simulink model "BD_CONV2"  (Simulink 4.1.1)
settings: Solver=ode1  SolverMode=SingleTasking  StartTime=0.0  StopTime=max(cyc_mph(:,1))  FixedStep=1  MaxStep=1  RelTol=1e-3  AbsTol=1e-3
undefined symbols (not defined in the file): cyc_mph, ess_on, ex_calc, fc_ct_trq, fc_emis, fc_inertia, fc_map_spd, fc_max_trq, fc_spd_scale, fc_trq_scale, fd_inertia, fd_loss, fd_ratio, gb_dnshift_load, gb_dnshift_spd, gb_gears_num, gb_inertia, gb_num_init, gb_ratio, gb_shift_delay, gb_spd_scale, gb_trq_scale, gb_upshift_load, gb_upshift_spd, logFlag, tx_eff_map, tx_map_spd, tx_map_trq, vc_clutch_bool, vc_idle_bool, vc_idle_spd, vc_key_on, vc_launch_spd, veh_air_density, veh_CD, veh_FA, veh_gravity, veh_mass, wh_axle_loss_mass, wh_axle_loss_trq, wh_front_active_bool, wh_inertia, wh_max_front_brake_force, wh_max_rear_brake_force, wh_radius, wh_rear_active_bool, wh_slip, wh_slip_force_coeff
libraries: lib_wheel2 x12, lib_drive_cycle2 x2, lib_accessory2 x2, lib_etc x2, lib_interactive x1, lib_exhaust x1, lib_fuel_converter3 x1, lib_help x1
(part 11 of 11)

== system BD_CONV2/<cs> control strategy/Clutch Control/Clutch Control/clutch control/gearbox speed estimator ==
  gb_spd_in_r if no gear change : Inport  Port=1  LatchInput=off
  Block NOTES : Subsystem
      settings: RTWFcnNameOpts=Auto  RTWFileNameOpts=Auto
      mask Display: disp('Block\nNOTES')
  Constant : Constant  Orientation=left  Value=eps
  Constant1 : Constant  Orientation=left  Value=0
  Constant2 : Constant  Orientation=left  Value=1
  Constant3 : Constant  Orientation=left  Value=0.11
  Gain : Gain  Gain=0.447  Multiplication=Element-wise(K.*u)  SaturateOnIntegerOverflow=on
  IC : InitialCondition  Value=cyc_mph(1,2)*0.447/wh_radius*fd_ratio*gb_ratio(gb_num_init)
  IC1 : InitialCondition  Value=1
  Logical : Logic  Operator=AND  Inputs=2
  Product : Product  Inputs=**/  Multiplication=Element-wise(.*)  SaturateOnIntegerOverflow=on
  Relational : RelationalOperator  Operator=>
  Relational1 : RelationalOperator  Operator=<=
  Sum : Sum  Inputs=++  SaturateOnIntegerOverflow=on
  Sum1 : Sum  Inputs=-+  SaturateOnIntegerOverflow=on
  Switch : Switch  Threshold=eps
  Switch1 : Switch  Threshold=eps
  dt : Subsystem
      settings: RTWFcnNameOpts=Auto  RTWFileNameOpts=Auto
  Out1 : Outport  Port=1
  wires:
  dt/1(Out1) -> Relational1/1
  Logical/1 -> Switch1/2
  IC1/1 -> Logical/1
  Relational1/1 -> Logical/2
  Constant3/1 -> Relational1/2
  [gb_spd_in_a] -> Product/1
  gb_spd_in_r if no gear change/1 -> Switch1/3
  Switch1/1 -> Out1/1
  Switch/1 -> IC/1
  Relational/1 -> IC1/1
  Sum1/1 -> Relational/1
  Constant2/1 -> Relational/2
  [mpha] -> Sum1/1, Gain/1
  [cyc_mph_r] -> Sum1/2
  Constant/1 -> Sum/2
  IC/1 -> Switch1/1
  Constant1/1 -> Switch/3
  [veh_spd_a_rec] -> Switch/2, Sum/1
  Gain/1 -> Product/2
  Sum/1 -> Product/3
  Product/1 -> Switch/1

== system BD_CONV2/<cs> control strategy/Fuel Converter Control conventional ic engine/conventional IC engine/Fuel Converter Control/key_on ==
  Clock : Clock
      settings: DisplayTime=off  Decimation=10
  Fcn1 : Fcn  Expr=rem(u[1],period)
  Look-Up Table : Lookup  InputValues=t  OutputValues=y
  out_1 : Outport  Port=1  InitialOutput=0
  wires:
  Fcn1/1 -> Look-Up Table/1
  Clock/1 -> Fcn1/1
  Look-Up Table/1 -> out_1/1

== system BD_CONV2/<cs> control strategy/Gearbox Control manual shift logic/manual shift logic/gearbox  control/Block NOTES ==
  note: This gearbox control block computes the current gear number given the gearbox's
      | req'd output torque and speed and an estimate its efficiency.  Upshifts occur, given a
      | certain engine speed,  when the estimated engine load falls below the upshift curve
      | in engine speed/load space, and downshifts likewise occur when estimated engine
      | load rises above the downshift curve.  Separate upshift and downshift curves are
      | defined for each gear.  An upshift may not be immediately followed by a downshift.
      | If the tires are about to slip, don't upshift unless the engine would be at max. speed.
      | Enforce this rule by setting the load to 1 when the tires are about to slip.

== system BD_CONV2/<cs> control strategy/Gearbox Control manual shift logic/manual shift logic/gearbox  control/allow downshift? ==
  prev gearnum : Inport  Port=1  LatchInput=off
  Logical Operator : Logic  Operator=NOR  Inputs=2
  Memory : Memory  X0=1  InheritSampleTime=off
      settings: RTWStateStorageClass=Auto
  Memory1 : Memory  X0=1  InheritSampleTime=off
      settings: RTWStateStorageClass=Auto
  Relational Operator1 : RelationalOperator  Operator=>
  Relational Operator2 : RelationalOperator  Operator=>
  allow shift : Outport  Port=1  InitialOutput=0
  wires:
  Logical Operator/1 -> allow shift/1
  prev gearnum/1 -> Relational Operator1/1, Memory/1, Relational Operator2/1
  Relational Operator1/1 -> Logical Operator/1
  Memory/1 -> Relational Operator1/2, Memory1/1
  Memory1/1 -> Relational Operator2/2
  Relational Operator2/1 -> Logical Operator/2

== system BD_CONV2/<cs> control strategy/Gearbox Control manual shift logic/manual shift logic/gearbox  control/downshift  command ==
  prev gear number : Inport  Port=1  LatchInput=off
  engine load : Inport  Port=2  LatchInput=off
  engine speed : Inport  Port=3  LatchInput=off
  Mux : Mux  Inputs=2
      settings: DisplayOption=none
  Relational Operator : RelationalOperator  Operator=>
  load fraction : Subsystem  mask(Gear Selector){spd=gb_dnshift_spd, load=gb_dnshift_load}
      mask prompts: spd "Speeds:"; load "Load Fractions:"
      mask help:
      | This block will perform a linear interplation (extrapolation outside of bounds) to determine the shift point load fraction associated with the current gear number and speed.
      |
      | The Speeds parameter should be defined as an array of vectors containing speeds for each gear number.  The Load Fractions parameter should be defined as a array of vectors containing load fractions indexed by the speeds in the Speeds parameter for each gear number.
      settings: RTWFcnNameOpts=Auto  RTWFileNameOpts=Auto
      mask Help:
      | Reference the base workspace variables - gb_**shift_spd and gb_**shift_load  where ** is either up for upshift conditions or dn for downshift conditions.
      | 
      | Or define the arrays as follows:
      | 
      | {[spd1 spd2 spd3 spd4]; [spd1 spd2 spd3 spd4]; ...}
      | 
      | {[load1 load2 load3 load4]; [load1 load2 load3 load4]; ...}
      | 
      | where each array contains one row for each gear in the gearbox.  Speeds should be defined in rad/s and loads as a decimal fraction.
  command : Outport  Port=1  InitialOutput=0
  wires:
  load fraction/1(Out1) -> Relational Operator/2
  Mux/1 -> load fraction/1(In1)
  engine load/1 -> Relational Operator/1
  prev gear number/1 -> Mux/1
  engine speed/1 -> Mux/2
  Relational Operator/1 -> command/1

== system BD_CONV2/<cs> control strategy/Gearbox Control manual shift logic/manual shift logic/gearbox  control/gearbox speed estimator ==
  gb_spd_in_r if no gear change : Inport  Port=1  LatchInput=off
  Block NOTES : Subsystem
      settings: RTWFcnNameOpts=Auto  RTWFileNameOpts=Auto
      mask Display: disp('Block\nNOTES')
  Constant : Constant  Orientation=left  Value=eps
  Constant1 : Constant  Orientation=left  Value=0
  Constant2 : Constant  Orientation=left  Value=1
  Constant3 : Constant  Orientation=left  Value=0.11
  Gain : Gain  Gain=0.447  Multiplication=Element-wise(K.*u)  SaturateOnIntegerOverflow=on
  IC : InitialCondition  Value=cyc_mph(1,2)*0.447/wh_radius*fd_ratio*gb_ratio(gb_num_init)
  IC1 : InitialCondition  Value=1
  Logical : Logic  Operator=AND  Inputs=2
  Product : Product  Inputs=**/  Multiplication=Element-wise(.*)  SaturateOnIntegerOverflow=on
  Relational : RelationalOperator  Operator=>
  Relational1 : RelationalOperator  Operator=<=
  Sum : Sum  Inputs=++  SaturateOnIntegerOverflow=on
  Sum1 : Sum  Inputs=-+  SaturateOnIntegerOverflow=on
  Switch : Switch  Threshold=eps
  Switch1 : Switch  Threshold=eps
  dt : Subsystem
      settings: RTWFcnNameOpts=Auto  RTWFileNameOpts=Auto
  Out1 : Outport  Port=1
  wires:
  Product/1 -> Switch/1
  Sum/1 -> Product/3
  Gain/1 -> Product/2
  [veh_spd_a_rec] -> Sum/1, Switch/2
  Constant1/1 -> Switch/3
  IC/1 -> Switch1/1
  Constant/1 -> Sum/2
  [cyc_mph_r] -> Sum1/2
  [mpha] -> Gain/1, Sum1/1
  Constant2/1 -> Relational/2
  Sum1/1 -> Relational/1
  Relational/1 -> IC1/1
  Switch/1 -> IC/1
  Switch1/1 -> Out1/1
  gb_spd_in_r if no gear change/1 -> Switch1/3
  [gb_spd_in_a] -> Product/1
  Constant3/1 -> Relational1/2
  Relational1/1 -> Logical/2
  IC1/1 -> Logical/1
  Logical/1 -> Switch1/2
  dt/1(Out1) -> Relational1/1

== system BD_CONV2/<cs> control strategy/Gearbox Control manual shift logic/manual shift logic/gearbox  control/shifting1 ==
  gear number : Inport  Port=1  LatchInput=off
  Constant : Constant  Value=gb_shift_delay-1e-6
  Relational Operator : RelationalOperator  Operator=<
  time since last shift : Subsystem
      settings: RTWFcnNameOpts=Auto  RTWFileNameOpts=Auto
      mask Display: disp('time since\nlast shift')
  out_1 : Outport  Port=1  InitialOutput=0
  wires:
  Relational Operator/1 -> out_1/1
  gear number/1 -> time since last shift/1(in_1)
  Constant/1 -> Relational Operator/2
  time since last shift/1(out_1) -> Relational Operator/1

== system BD_CONV2/<cs> control strategy/Gearbox Control manual shift logic/manual shift logic/gearbox  control/upshift  command ==
  prev gear number : Inport  Port=1  LatchInput=off
  engine load : Inport  Port=2  LatchInput=off
  engine speed : Inport  Port=3  LatchInput=off
  Mux : Mux  Inputs=2
      settings: DisplayOption=none
  Relational Operator : RelationalOperator  Operator=<
  load fraction : Subsystem  mask(Gear Selector){spd=gb_upshift_spd, load=gb_upshift_load}
      mask prompts: spd "Speeds:"; load "Load Fractions:"
      mask help:
      | This block will perform a linear interplation (extrapolation outside of bounds) to determine the shift point load fraction associated with the current gear number and speed.
      |
      | The Speeds parameter should be defined as an array of vectors containing speeds for each gear number.  The Load Fractions parameter should be defined as a array of vectors containing load fractions indexed by the speeds in the Speeds parameter for each gear number.
      settings: RTWFcnNameOpts=Auto  RTWFileNameOpts=Auto
      mask Help:
      | Reference the base workspace variables - gb_**shift_spd and gb_**shift_load  where ** is either up for upshift conditions or dn for downshift conditions.
      | 
      | Or define the arrays as follows:
      | 
      | {[spd1 spd2 spd3 spd4]; [spd1 spd2 spd3 spd4]; ...}
      | 
      | {[load1 load2 load3 load4]; [load1 load2 load3 load4]; ...}
      | 
      | where each array contains one row for each gear in the gearbox.  Speeds should be defined in rad/s and loads as a decimal fraction.
  command : Outport  Port=1  InitialOutput=0
  wires:
  load fraction/1(Out1) -> Relational Operator/2
  engine load/1 -> Relational Operator/1
  prev gear number/1 -> Mux/1
  Mux/1 -> load fraction/1(In1)
  engine speed/1 -> Mux/2
  Relational Operator/1 -> command/1

== system BD_CONV2/ACC MECH <accm>/mechanical accessory model and interface/Mechanical Accessory model/backward model/enhancedToWorkspace ==
  In1 : Inport  Port=1  LatchInput=off
  To Workspace : ToWorkspace  VariableName=acc_mech_pwr_r  SampleTime=-1  SaveFormat=Array
  wires:
  In1/1 -> To Workspace/1

== system BD_CONV2/ACC MECH <accm>/mechanical accessory model and interface/Mechanical Accessory model/backward model/enhancedToWorkspace1 ==
  In1 : Inport  Port=1  LatchInput=off
  To Workspace : ToWorkspace  VariableName=acc_mech_trq_r  SampleTime=-1  SaveFormat=Array
  wires:
  In1/1 -> To Workspace/1

== system BD_CONV2/ACC MECH <accm>/mechanical accessory model and interface/Mechanical Accessory model/backward model/mechanical accessories (Nm) ==
  w_APU : Inport  Port=1  LatchInput=off
  Mechanical Accessories: Const Mech Var Elect : lib_accessory2/ACC MECH models/Mechanical Accessories: Const Mech Var Elect
  T_acc : Outport  Port=1
  P_mech_acc : Outport  Port=2
  wires:
  w_APU/1 -> Mechanical Accessories: Const Mech Var Elect/1
  Mechanical Accessories: Const Mech Var Elect/1 -> T_acc/1
  Mechanical Accessories: Const Mech Var Elect/2 -> P_mech_acc/1

== system BD_CONV2/fuel converter <fc>/IC Engine Model  &  Interface/ic engine model/engine speed estimator/Block NOTES ==
  note: If the clutch is engaged and the trace was missed in the previous time step:
      | The estimated engine speed for the current time step is the actual engine
      | speed from the previous time step.
      |
      | If the clutch is disengaged and the speed is commanded to increase (spin up):
      | The engine speed is the lesser of the commanded speed and the maximum
      | speed attainable given the engine capability.
      |
      | If the clutch is disengaged at the speed is commanded to decrease (spin down):
      | The engine speed is computed by integrating with respect to time the ratio of
      |  closed-throttle torque to engine inertia.
      |
      | Otherwise:
      | The engine speed is equal to the speed command, but no greater than the
      | engine's maximum speed nor less than the engine's idle speed (if the engine is on.)

== system BD_CONV2/fuel converter <fc>/IC Engine Model  &  Interface/ic engine model/engine speed estimator/dt ==
  Clock : Clock
      settings: DisplayTime=off  Decimation=10
  Memory1 : Memory  X0=-0.1  InheritSampleTime=off
      settings: RTWStateStorageClass=Auto
  Sum1 : Sum  Inputs=+-  SaturateOnIntegerOverflow=on
  out_1 : Outport  Port=1  InitialOutput=0
  wires:
  Clock/1 -> Sum1/1, Memory1/1
  Memory1/1 -> Sum1/2
  Sum1/1 -> out_1/1

== system BD_CONV2/fuel converter <fc>/IC Engine Model  &  Interface/ic engine model/engine speed estimator/effect of inertia (Nm) ==
  req'd spd (rad/s) : Inport  Port=1  LatchInput=off
  prev spd : Inport  Port=2  LatchInput=off
  Clock : Clock
      settings: DisplayTime=off  Decimation=10
  Constant : Constant  Value=fc_inertia
  Memory : Memory  X0=-0.1  InheritSampleTime=off
      settings: RTWStateStorageClass=Auto
  Product1 : Product  Inputs=**/  Multiplication=Element-wise(.*)  SaturateOnIntegerOverflow=on
  Sum : Sum  Inputs=+-  SaturateOnIntegerOverflow=on
  Sum1 : Sum  Inputs=+-  SaturateOnIntegerOverflow=on
  (Nm) : Outport  Port=1  InitialOutput=0
  wires:
  Constant/1 -> Product1/1
  Clock/1 -> Sum1/1, Memory/1
  Memory/1 -> Sum1/2
  Product1/1 -> (Nm)/1
  prev spd/1 -> Sum/2
  req'd spd (rad/s)/1 -> Sum/1
  Sum1/1 -> Product1/3
  Sum/1 -> Product1/2

== system BD_CONV2/fuel converter <fc>/IC Engine Model  &  Interface/ic engine model/engine speed estimator/just started spin-down/spin-up ==
  state : Inport  Port=1  LatchInput=off
  Logical Operator : Logic  Operator=AND  Inputs=2
  Logical Operator1 : Logic  Operator=NOT  Inputs=1
  Memory1 : Memory  X0=1  InheritSampleTime=off
      settings: RTWStateStorageClass=Auto
  trigger : Outport  Port=1  InitialOutput=0
  wires:
  state/1 -> Memory1/1, Logical Operator/1
  Logical Operator/1 -> trigger/1
  Logical Operator1/1 -> Logical Operator/2
  Memory1/1 -> Logical Operator1/1

== system BD_CONV2/fuel converter <fc>/IC Engine Model  &  Interface/ic engine model/engine speed estimator/no-lag Reset Integrator ==
  in_1 : Inport  Port=1  LatchInput=off
  in_2 : Inport  Port=2  LatchInput=off
  in_3 : Inport  Port=3  LatchInput=off
  Constant : Constant  Value=0
  Memory : Memory  Orientation=left  X0=initval  InheritSampleTime=off
      settings: RTWStateStorageClass=Auto
  Product : Product  Inputs=2  Multiplication=Element-wise(.*)  SaturateOnIntegerOverflow=on
  Sum : Sum  Inputs=++  SaturateOnIntegerOverflow=on
  Switch : Switch  Threshold=eps
  dt : Subsystem  Orientation=down
      settings: RTWFcnNameOpts=Auto  RTWFileNameOpts=Auto
  in_2==0 : RelationalOperator  Operator===
  out_1 : Outport  Port=1  InitialOutput=0
  wires:
  Constant/1 -> in_2==0/2
  in_2==0/1 -> Switch/2
  Switch/1 -> Memory/1, out_1/1
  Sum/1 -> Switch/1
  Memory/1 -> Sum/1
  Product/1 -> Sum/2
  dt/1(out_1) -> Product/1
  in_1/1 -> Product/2
  in_2/1 -> in_2==0/1
  in_3/1 -> Switch/3

== system BD_CONV2/fuel converter <fc>/IC Engine Model  &  Interface/ic engine model/engine torque/Block NOTES ==
  note: If the engine is not spinning down with the clutch disengaged:
      | 1.  Engine brake (aka map) torque is given by the required shaft
      | torque plus enough torque to accelerate the engine's rotating
      | parts as commanded and torque to power the accessories,
      | subject to the engine's torque limits at the current speed.
      | 2.  Shaft torque is engine brake torque less the effects of inertia
      | and accessories.
      |
      | If the engine is spinning down:
      | 1.  Engine brake/map torque is the closed-throttle torque.
      | 2.  Shaft torque is zero.

== system BD_CONV2/fuel converter <fc>/IC Engine Model  &  Interface/ic engine model/engine torque/T_closed throttle ==
  w_APU : Inport  Port=1  LatchInput=off
  Saturation : Saturate  UpperLimit=max(fc_map_spd)*fc_spd_scale  LowerLimit=min(fc_map_spd)*fc_spd_scale  LinearizeAsGain=on
  ctt lookup : Lookup  InputValues=fc_map_spd*fc_spd_scale  OutputValues=fc_ct_trq*fc_trq_scale
  T_closed throttle : Outport  Port=1  InitialOutput=0
  wires:
  ctt lookup/1 -> T_closed throttle/1
  Saturation/1 -> ctt lookup/1
  w_APU/1 -> Saturation/1

== system BD_CONV2/fuel converter <fc>/IC Engine Model  &  Interface/ic engine model/engine torque/T_max ==
  w_APU : Inport  Port=1  LatchInput=off
  Saturation1 : Saturate  UpperLimit=max(fc_map_spd)*fc_spd_scale  LowerLimit=min(fc_map_spd)*fc_spd_scale  LinearizeAsGain=on
  max_torque lookup : Lookup  InputValues=fc_map_spd*fc_spd_scale  OutputValues=fc_max_trq*fc_trq_scale
  T_max : Outport  Port=1  InitialOutput=0
  tag scope: engine_speed=scoped
  wires:
  w_APU/1 -> Saturation1/1
  max_torque lookup/1 -> T_max/1
  Saturation1/1 -> max_torque lookup/1, [engine_speed]

== system BD_CONV2/fuel converter <fc>/IC Engine Model  &  Interface/ic engine model/engine torque/effect of inertia (Nm) ==
  engine spd (rad/s) : Inport  Port=1  LatchInput=off
  >=0 : Saturate  UpperLimit=inf  LowerLimit=0  LinearizeAsGain=on
  Block NOTES : Subsystem
      settings: RTWFcnNameOpts=Auto  RTWFileNameOpts=Auto
      mask Display: disp('Block\nNOTES')
  Clock : Clock
      settings: DisplayTime=off  Decimation=10
  Constant : Constant  Orientation=left  Value=fc_inertia
  Constant1 : Constant  Value=max(fc_max_trq)*fc_trq_scale
  Constant2 : Constant  Orientation=left  Value=0.01
  Memory : Memory  X0=-0.1  InheritSampleTime=off
      settings: RTWStateStorageClass=Auto
  Memory1 : Memory  X0=vc_idle_spd*vc_key_on(1,2)  InheritSampleTime=off
      settings: RTWStateStorageClass=Auto
  MinMax : MinMax  Function=min  Inputs=2
  Product : Product  Inputs=2  Multiplication=Element-wise(.*)  SaturateOnIntegerOverflow=on
  Product1 : Product  Inputs=*/*  Multiplication=Element-wise(.*)  SaturateOnIntegerOverflow=on
  Relational : RelationalOperator  Operator=>
  Sum : Sum  Inputs=+-  SaturateOnIntegerOverflow=on
  Sum1 : Sum  Inputs=+-  SaturateOnIntegerOverflow=on
  Sum2 : Sum  Inputs=-+  SaturateOnIntegerOverflow=on
  Switch : Switch  Threshold=eps
  engine inertia as a function of total vehicle inertia (generous approximation) : Subsystem  Orientation=down
      settings: RTWFcnNameOpts=Auto  RTWFileNameOpts=Auto
  (Nm) : Outport  Port=1  InitialOutput=0
  wires:
  Sum/1 -> >=0/1, Switch/3
  Memory1/1 -> Sum/2
  Product/1 -> MinMax/1
  Constant1/1 -> Product/2
  engine inertia as a function of total vehicle inertia (generous approximation)/1(Out1) -> Product/1
  Product1/1 -> MinMax/2
  MinMax/1 -> (Nm)/1
  [cyc_mph_r_prev] -> Sum2/2
  [mpha_prev] -> Sum2/1
  Switch/1 -> Product1/1
  Sum1/1 -> Product1/2
  Constant/1 -> Product1/3
  Memory/1 -> Sum1/2
  Clock/1 -> Memory/1, Sum1/1
  Relational/1 -> Switch/2
  >=0/1 -> Switch/1
  Sum2/1 -> Relational/1
  Constant2/1 -> Relational/2
  engine spd (rad/s)/1 -> Memory1/1, Sum/1

== system BD_CONV2/gearbox <gb> old/gearbox model & interface/gearbox model/Pout/Pin neglecting inertia/Pout/Pin (neglecting inertia) ==
  in_1 : Inport  Port=1  LatchInput=off
  in_2 : Inport  Port=2  LatchInput=off
  Fcn : Fcn  Expr=1/u
  Product : Product  Inputs=2  Multiplication=Element-wise(.*)  SaturateOnIntegerOverflow=on
  out_1 : Outport  Port=1  InitialOutput=0
  wires:
  in_1/1 -> Product/1
  Fcn/1 -> Product/2
  Product/1 -> out_1/1
  in_2/1 -> Fcn/1

== system BD_CONV2/gearbox <gb> old/gearbox model & interface/gearbox model/Pout/Pin neglecting inertia/make division bombproof ==
  note: only add eps if Tin-Tinertia is == 0 (this avoids problems when Tin-Tineratia == -eps
      | which happens from time to time
  Tin-Tinertia : Inport  Port=1  LatchInput=off
  Block NOTES : Subsystem
      settings: RTWFcnNameOpts=Auto  RTWFileNameOpts=Auto
      mask Display: disp('Block\nNOTES')
  Constant : Constant  Orientation=up  Value=eps
  Constant1 : Constant  Orientation=up  Value=0
  Product : Product  Inputs=2  Multiplication=Element-wise(.*)  SaturateOnIntegerOverflow=on
  Relational Operator1 : RelationalOperator  Operator===
  make division bombproof : Sum  Inputs=++  SaturateOnIntegerOverflow=on
  Out1 : Outport  Port=1
  wires:
  Tin-Tinertia/1 -> make division bombproof/1, Relational Operator1/1
  Constant1/1 -> Relational Operator1/2
  Product/1 -> make division bombproof/2
  Relational Operator1/1 -> Product/1
  Constant/1 -> Product/2
  make division bombproof/1 -> Out1/1

== system BD_CONV2/gearbox <gb> old/gearbox model & interface/gearbox model/gearbox controller interface/enhancedToWorkspace1 ==
  In1 : Inport  Port=1  LatchInput=off
  To Workspace : ToWorkspace  VariableName=gb_gear_ratio  SampleTime=-1  SaveFormat=Array
  wires:
  In1/1 -> To Workspace/1

== system BD_CONV2/gearbox <gb> old/gearbox model & interface/gearbox model/gearbox controller interface/enhancedToWorkspace8 ==
  In1 : Inport  Port=1  LatchInput=off
  To Workspace : ToWorkspace  VariableName=gb_shifting  SampleTime=-1  SaveFormat=Array
  wires:
  In1/1 -> To Workspace/1

== system BD_CONV2/gearbox <gb> old/gearbox model & interface/gearbox model/loss (Nm)/3D discrete lookup table (sfun) ==
  lookup speed (rad/s) : Inport  Port=1  LatchInput=off
  lookup trq (Nm) : Inport  Port=2  LatchInput=off
  "gear_number  (e.g., 1, 2, 3)" : Inport  Port=3  LatchInput=off
  Mux : Mux  Inputs=3
  Saturation : Saturate  UpperLimit=max(tx_map_spd)  LowerLimit=min(tx_map_spd)  LinearizeAsGain=on
  Saturation1 : Saturate  UpperLimit=max(tx_map_trq)  LowerLimit=min(tx_map_trq)  LinearizeAsGain=on
  Saturation2 : Saturate  UpperLimit=size(tx_eff_map,3)  LowerLimit=1  LinearizeAsGain=on
  discrete interp2d : S-Function  FunctionName=sfun_discreteLookup3d  Parameters=tx_map_trq, tx_map_spd, tx_eff_map  PortCounts=[]  SFunctionModules=''
  tx_eff : Outport  Port=1
  wires:
  Saturation2/1 -> Mux/3
  "gear_number  (e.g., 1, 2, 3)"/1 -> Saturation2/1
  Saturation1/1 -> Mux/2
  lookup trq (Nm)/1 -> Saturation1/1
  Saturation/1 -> Mux/1
  lookup speed (rad/s)/1 -> Saturation/1
  Mux/1 -> discrete interp2d/1
  discrete interp2d/1 -> tx_eff/1

== system BD_CONV2/gearbox <gb> old/gearbox model & interface/gearbox model/loss (Nm)/Block NOTES ==
  note: Revision Notes:
  note: 09/20/02:tm modifed lower input to switch after T_loss_at_input to pass the
      | total torque input as the loss when tx_eff=0
      | 5 July 2001:mpo changing loss block to a lookup table methodology
      | 12/20/00:tm revised loss saturation block. lower limit changed
      | from 1 to 0 and upper limit changed from 100 to inf to prevent over or under penalties

== system BD_CONV2/gearbox <gb> old/gearbox model & interface/gearbox model/loss (Nm)/enhancedToWorkspace ==
  In1 : Inport  Port=1  LatchInput=off
  To Workspace : ToWorkspace  VariableName=gb_current_gear_ratio  SampleTime=-1  SaveFormat=Array
  wires:
  In1/1 -> To Workspace/1

== system BD_CONV2/vehicle, wheel, & axle front/rear <wh> 2 axle --> 1 driveline/models and interface/vehicle <veh>/power logging--achieved/Joules ==
  In1 : Inport  Port=1  LatchInput=off
  To Workspace : ToWorkspace  VariableName=veh_energy_a  SampleTime=-1  SaveFormat=Array
  wires:
  In1/1 -> To Workspace/1

== system BD_CONV2/vehicle, wheel, & axle front/rear <wh> 2 axle --> 1 driveline/models and interface/vehicle <veh>/power logging--achieved/horse power ==
  In1 : Inport  Port=1  LatchInput=off
  To Workspace : ToWorkspace  VariableName=veh_pwr_a_hp  SampleTime=-1  SaveFormat=Array
  wires:
  In1/1 -> To Workspace/1

== system BD_CONV2/vehicle, wheel, & axle front/rear <wh> 2 axle --> 1 driveline/models and interface/vehicle <veh>/power logging--achieved/watts ==
  In1 : Inport  Port=1  LatchInput=off
  To Workspace : ToWorkspace  VariableName=veh_pwr_a  SampleTime=-1  SaveFormat=Array
  wires:
  In1/1 -> To Workspace/1

== system BD_CONV2/vehicle, wheel, & axle front/rear <wh> 2 axle --> 1 driveline/models and interface/vehicle <veh>/power logging--request/Joules ==
  In1 : Inport  Port=1  LatchInput=off
  To Workspace : ToWorkspace  VariableName=veh_energy_r  SampleTime=-1  SaveFormat=Array
  wires:
  In1/1 -> To Workspace/1

== system BD_CONV2/vehicle, wheel, & axle front/rear <wh> 2 axle --> 1 driveline/models and interface/vehicle <veh>/power logging--request/horse power ==
  In1 : Inport  Port=1  LatchInput=off
  To Workspace : ToWorkspace  VariableName=veh_pwr_r_hp  SampleTime=-1  SaveFormat=Array
  wires:
  In1/1 -> To Workspace/1

== system BD_CONV2/vehicle, wheel, & axle front/rear <wh> 2 axle --> 1 driveline/models and interface/vehicle <veh>/power logging--request/watts ==
  In1 : Inport  Port=1  LatchInput=off
  To Workspace : ToWorkspace  VariableName=veh_pwr_r  SampleTime=-1  SaveFormat=Array
  wires:
  In1/1 -> To Workspace/1

== system BD_CONV2/vehicle, wheel, & axle front/rear <wh> 2 axle --> 1 driveline/models and interface/vehicle <veh>/record achieved force outputs/enhancedToWorkspace ==
  In1 : Inport  Port=1  LatchInput=off
  To Workspace : ToWorkspace  VariableName=veh_pwr_accel_a  SampleTime=-1  SaveFormat=Array
  wires:
  In1/1 -> To Workspace/1

== system BD_CONV2/vehicle, wheel, & axle front/rear <wh> 2 axle --> 1 driveline/models and interface/vehicle <veh>/record achieved force outputs/enhancedToWorkspace1 ==
  In1 : Inport  Port=1  LatchInput=off
  To Workspace : ToWorkspace  VariableName=veh_pwr_drag_a  SampleTime=-1  SaveFormat=Array
  wires:
  In1/1 -> To Workspace/1

== system BD_CONV2/vehicle, wheel, & axle front/rear <wh> 2 axle --> 1 driveline/models and interface/vehicle <veh>/record achieved force outputs/enhancedToWorkspace2 ==
  In1 : Inport  Port=1  LatchInput=off
  To Workspace : ToWorkspace  VariableName=veh_pwr_ascent_a  SampleTime=-1  SaveFormat=Array
  wires:
  In1/1 -> To Workspace/1

== system BD_CONV2/vehicle, wheel, & axle front/rear <wh> 2 axle --> 1 driveline/models and interface/vehicle <veh>/record achieved force outputs/enhancedToWorkspace3 ==
  In1 : Inport  Port=1  LatchInput=off
  To Workspace : ToWorkspace  VariableName=veh_pwr_rr_a  SampleTime=-1  SaveFormat=Array
  wires:
  In1/1 -> To Workspace/1

== system BD_CONV2/vehicle, wheel, & axle front/rear <wh> 2 axle --> 1 driveline/models and interface/vehicle <veh>/record achieved force outputs/rolling resistance force ==
  average vehicle speed over time step (m/s) : Inport  Port=1  LatchInput=off
  force req'd to overcome rolling resistance (N) : lib_wheel2/Submodels/force req'd to overcome rolling resistance (N)
      settings: RTWFcnNameOpts=Auto  RTWFileNameOpts=Auto
  Fr (N) : Outport  Port=1
  wires:
  average vehicle speed over time step (m/s)/1 -> force req'd to overcome rolling resistance (N)/1
  force req'd to overcome rolling resistance (N)/1 -> Fr (N)/1

== system BD_CONV2/vehicle, wheel, & axle front/rear <wh> 2 axle --> 1 driveline/models and interface/wheel and axle  front/rear <wh>/front force/brake request  controller interface ==
  F_front_brake_req : Outport  Port=1  InitialOutput=0
  wires:
  [F_front_brake_req] -> F_front_brake_req/1

== system BD_CONV2/vehicle, wheel, & axle front/rear <wh> 2 axle --> 1 driveline/models and interface/wheel and axle  front/rear <wh>/front force/enhancedToWorkspace11 ==
  In1 : Inport  Port=1  LatchInput=off
  To Workspace : ToWorkspace  VariableName=wh_front_brake_r  SampleTime=-1  SaveFormat=Array
  wires:
  In1/1 -> To Workspace/1

== system BD_CONV2/vehicle, wheel, & axle front/rear <wh> 2 axle --> 1 driveline/models and interface/wheel and axle  front/rear <wh>/limits and losses diagnostics/enhancedToWorkspace ==
  In1 : Inport  Port=1  LatchInput=off
  To Workspace : ToWorkspace  VariableName=wh_brake_loss_pwr  SampleTime=-1  SaveFormat=Array
  wires:
  In1/1 -> To Workspace/1

== system BD_CONV2/vehicle, wheel, & axle front/rear <wh> 2 axle --> 1 driveline/models and interface/wheel and axle  front/rear <wh>/rear force/brake request controller interface1 ==
  F_rear_brake_req : Outport  Port=1  InitialOutput=0
  wires:
  [F_rear_brake_req] -> F_rear_brake_req/1

== system BD_CONV2/vehicle, wheel, & axle front/rear <wh> 2 axle --> 1 driveline/models and interface/wheel and axle  front/rear <wh>/rear force/enhancedToWorkspace ==
  In1 : Inport  Port=1  LatchInput=off
  To Workspace : ToWorkspace  VariableName=wh_rear_brake_r  SampleTime=-1  SaveFormat=Array
  wires:
  In1/1 -> To Workspace/1

== system BD_CONV2/vehicle, wheel, & axle front/rear <wh> 2 axle --> 1 driveline/models and interface/wheel and axle  front/rear <wh>/tire slip model (m/s)/Block NOTES ==
  note: This block implements the effects of finite tire slip (with respect to the road) on the
      | vehicle speed/wheel speed relationship.  Slip is defined as s=(omega*r - v) / v.  The
      | one-to-one mapping of slip to normalized tractive force, F_tract/W_front_axle, up to
      | the maximum, is stored in the variables "wh_slip" and "wh_slip_force_coeff."  The
      | slip calculation here is overridden if the actual axle speed and the requested axle
      | speed are the same, indicating that no drivetrain speed limits were encountered.

== system BD_CONV2/vehicle, wheel, & axle front/rear <wh> 2 axle --> 1 driveline/models and interface/wheel and axle  front/rear <wh>/tire slip model (m/s)/front axle ==
  In1 : Inport  Port=1  LatchInput=off
  In2 : Inport  Port=2  LatchInput=off
  Abs : Abs  SaturateOnIntegerOverflow=on
  Constant3 : Constant  Orientation=up  Value=0
  F/W : Product  Inputs=*/  Multiplication=Element-wise(.*)  SaturateOnIntegerOverflow=on
  Product : Product  Inputs=2  Multiplication=Element-wise(.*)  SaturateOnIntegerOverflow=on
  Relational Operator : RelationalOperator  Orientation=up  Operator=~=
  Saturation : Saturate  UpperLimit=max(wh_slip_force_coeff)  LowerLimit=min(wh_slip_force_coeff)  LinearizeAsGain=on
  Sign : Signum
  Switch : Switch  Threshold=0
  s=s(F/W) : Lookup  InputValues=wh_slip_force_coeff  OutputValues=wh_slip
  Out1 : Outport  Port=1
  wires:
  Product/1 -> Out1/1
  In1/1 -> F/W/2
  In2/1 -> Sign/1, Abs/1
  s=s(F/W)/1 -> Product/1
  Sign/1 -> Product/2
  F/W/1 -> Switch/1
  Switch/1 -> Saturation/1
  Saturation/1 -> s=s(F/W)/1
  Abs/1 -> Relational Operator/1, F/W/1
  Relational Operator/1 -> Switch/2
  Constant3/1 -> Relational Operator/2, Switch/3

== system BD_CONV2/vehicle, wheel, & axle front/rear <wh> 2 axle --> 1 driveline/models and interface/wheel and axle  front/rear <wh>/tire slip model (m/s)/rear axle ==
  In1 : Inport  Port=1  LatchInput=off
  In2 : Inport  Port=2  LatchInput=off
  Abs : Abs  SaturateOnIntegerOverflow=on
  Constant3 : Constant  Orientation=up  Value=0
  F/W : Product  Inputs=*/  Multiplication=Element-wise(.*)  SaturateOnIntegerOverflow=on
  Product : Product  Inputs=2  Multiplication=Element-wise(.*)  SaturateOnIntegerOverflow=on
  Relational Operator : RelationalOperator  Orientation=up  Operator=~=
  Saturation : Saturate  UpperLimit=max(wh_slip_force_coeff)  LowerLimit=min(wh_slip_force_coeff)  LinearizeAsGain=on
  Sign : Signum
  Switch : Switch  Threshold=0
  s=s(F/W) : Lookup  InputValues=wh_slip_force_coeff  OutputValues=wh_slip
  Out1 : Outport  Port=1
  wires:
  Product/1 -> Out1/1
  In1/1 -> F/W/2
  In2/1 -> Sign/1, Abs/1
  s=s(F/W)/1 -> Product/1
  Sign/1 -> Product/2
  F/W/1 -> Switch/1
  Switch/1 -> Saturation/1
  Saturation/1 -> s=s(F/W)/1
  Abs/1 -> Relational Operator/1, F/W/1
  Relational Operator/1 -> Switch/2
  Constant3/1 -> Relational Operator/2, Switch/3

== system BD_CONV2/vehicle, wheel, & axle front/rear <wh> 2 axle --> 1 driveline/models and interface/wheel and axle  front/rear <wh>/tire slip model (rad/s)/enhancedToWorkspace ==
  In1 : Inport  Port=1  LatchInput=off
  To Workspace : ToWorkspace  VariableName=wh_slip_r  SampleTime=-1  SaveFormat=Array
  wires:
  In1/1 -> To Workspace/1

== system BD_CONV2/vehicle, wheel, & axle front/rear <wh> 2 axle --> 1 driveline/models and interface/wheel and axle  front/rear <wh>/tire slip model (rad/s)/front slip ==
  In1 : Inport  Port=1  LatchInput=off
  In2 : Inport  Port=2  LatchInput=off
  Abs : Abs  SaturateOnIntegerOverflow=on
  F/W : Product  Inputs=*/  Multiplication=Element-wise(.*)  SaturateOnIntegerOverflow=on
  Product : Product  Inputs=2  Multiplication=Element-wise(.*)  SaturateOnIntegerOverflow=on
  Saturation : Saturate  UpperLimit=max(wh_slip_force_coeff)  LowerLimit=min(wh_slip_force_coeff)  LinearizeAsGain=on
  Sign : Signum
  s=s(F/W) : Lookup  InputValues=wh_slip_force_coeff  OutputValues=wh_slip
  Out1 : Outport  Port=1
  wires:
  Product/1 -> Out1/1
  In1/1 -> F/W/2
  s=s(F/W)/1 -> Product/1
  In2/1 -> Sign/1, Abs/1
  Sign/1 -> Product/2
  Abs/1 -> F/W/1
  F/W/1 -> Saturation/1
  Saturation/1 -> s=s(F/W)/1

== system BD_CONV2/vehicle, wheel, & axle front/rear <wh> 2 axle --> 1 driveline/models and interface/wheel and axle  front/rear <wh>/tire slip model (rad/s)/rear slip ==
  In1 : Inport  Port=1  LatchInput=off
  In2 : Inport  Port=2  LatchInput=off
  Abs : Abs  SaturateOnIntegerOverflow=on
  F/W : Product  Inputs=*/  Multiplication=Element-wise(.*)  SaturateOnIntegerOverflow=on
  Product : Product  Inputs=2  Multiplication=Element-wise(.*)  SaturateOnIntegerOverflow=on
  Saturation : Saturate  UpperLimit=max(wh_slip_force_coeff)  LowerLimit=min(wh_slip_force_coeff)  LinearizeAsGain=on
  Sign : Signum
  s=s(F/W) : Lookup  InputValues=wh_slip_force_coeff  OutputValues=wh_slip
  Out1 : Outport  Port=1
  wires:
  Product/1 -> Out1/1
  In1/1 -> F/W/2
  s=s(F/W)/1 -> Product/1
  In2/1 -> Sign/1, Abs/1
  Sign/1 -> Product/2
  Abs/1 -> F/W/1
  F/W/1 -> Saturation/1
  Saturation/1 -> s=s(F/W)/1

== system BD_CONV2/<cs> control strategy/Clutch Control/Clutch Control/clutch control/gearbox speed estimator/Block NOTES ==
  note: The requested engine speed is replaced by an estimate of the
      | engine's previous speed whenever the vehicle missed the trace
      |  by more than 1 mph on the last time step.

== system BD_CONV2/<cs> control strategy/Clutch Control/Clutch Control/clutch control/gearbox speed estimator/dt ==
  Clock : Clock
      settings: DisplayTime=off  Decimation=10
  Memory1 : Memory  X0=-1  InheritSampleTime=off
      settings: RTWStateStorageClass=Auto
  Sum4 : Sum  Inputs=+-  SaturateOnIntegerOverflow=on
  Out1 : Outport  Port=1  InitialOutput=0
  wires:
  Clock/1 -> Sum4/1, Memory1/1
  Memory1/1 -> Sum4/2
  Sum4/1 -> Out1/1

== system BD_CONV2/<cs> control strategy/Gearbox Control manual shift logic/manual shift logic/gearbox  control/downshift  command/load fraction ==
  In1 : Inport  Port=1  LatchInput=off
  S-Function : S-Function  FunctionName=sfun_gearbox  Parameters=load, spd  PortCounts=[]  SFunctionModules=''
  Out1 : Outport  Port=1  InitialOutput=0
  wires:
  In1/1 -> S-Function/1
  S-Function/1 -> Out1/1

== system BD_CONV2/<cs> control strategy/Gearbox Control manual shift logic/manual shift logic/gearbox  control/gearbox speed estimator/Block NOTES ==
  note: The requested engine speed is replaced by an estimate of the
      | engine's previous speed whenever the vehicle missed the trace
      |  by more than 1 mph on the last time step.

== system BD_CONV2/<cs> control strategy/Gearbox Control manual shift logic/manual shift logic/gearbox  control/gearbox speed estimator/dt ==
  Clock : Clock
      settings: DisplayTime=off  Decimation=10
  Memory1 : Memory  X0=-1  InheritSampleTime=off
      settings: RTWStateStorageClass=Auto
  Sum4 : Sum  Inputs=+-  SaturateOnIntegerOverflow=on
  Out1 : Outport  Port=1  InitialOutput=0
  wires:
  Sum4/1 -> Out1/1
  Memory1/1 -> Sum4/2
  Clock/1 -> Memory1/1, Sum4/1

== system BD_CONV2/<cs> control strategy/Gearbox Control manual shift logic/manual shift logic/gearbox  control/shifting1/time since last shift ==
  in_1 : Inport  Port=1  LatchInput=off
  just shifted : Subsystem
      settings: RTWFcnNameOpts=Auto  RTWFileNameOpts=Auto
      mask Display: disp('just\nshifted')
  timer : Subsystem
      settings: RTWFcnNameOpts=Auto  RTWFileNameOpts=Auto
      mask Display: disp('timer')
  out_1 : Outport  Port=1  InitialOutput=0
  wires:
  in_1/1 -> just shifted/1(in_1)
  just shifted/1(out_1) -> timer/1(trigger)
  timer/1(time) -> out_1/1

== system BD_CONV2/<cs> control strategy/Gearbox Control manual shift logic/manual shift logic/gearbox  control/upshift  command/load fraction ==
  In1 : Inport  Port=1  LatchInput=off
  S-Function : S-Function  FunctionName=sfun_gearbox  Parameters=load, spd  PortCounts=[]  SFunctionModules=''
  Out1 : Outport  Port=1  InitialOutput=0
  wires:
  In1/1 -> S-Function/1
  S-Function/1 -> Out1/1

== system BD_CONV2/fuel converter <fc>/IC Engine Model  &  Interface/ic engine model/engine speed estimator/no-lag Reset Integrator/dt ==
  Clock : Clock
      settings: DisplayTime=off  Decimation=10
  Memory1 : Memory  X0=-0.1  InheritSampleTime=off
      settings: RTWStateStorageClass=Auto
  Sum1 : Sum  Inputs=+-  SaturateOnIntegerOverflow=on
  out_1 : Outport  Port=1  InitialOutput=0
  wires:
  Sum1/1 -> out_1/1
  Memory1/1 -> Sum1/2
  Clock/1 -> Memory1/1, Sum1/1

== system BD_CONV2/fuel converter <fc>/IC Engine Model  &  Interface/ic engine model/engine torque/effect of inertia (Nm)/Block NOTES ==
  note: Torque required to accelerate the engine inertia is taken from the engine
      | acceleration, and is assumed to be no less than zero if the trace was missed
      | at all on the previous time step.
      |
      | The torque required to accelerate the engine's inertia is never assumed to
      | be more than the product of the engine's maximum torque and the engine's
      | contribution to the total vehicle inertia.

== system BD_CONV2/fuel converter <fc>/IC Engine Model  &  Interface/ic engine model/engine torque/effect of inertia (Nm)/engine inertia as a function of total vehicle inertia (generous approximation) ==
  Product : Product  Orientation=down  Inputs=*/  Multiplication=Element-wise(.*)  SaturateOnIntegerOverflow=on
  Sum : Sum  Orientation=down  Inputs=++|  SaturateOnIntegerOverflow=on
  engine inertia as a fraction of total vehicle inertia  (generous approximation)--denomenator : Fcn  Orientation=down  Expr=fc_inertia*(u*fd_ratio/wh_radius)^2
  engine inertia as a fraction of total vehicle inertia  (generous approximation)--numerator : Fcn  Orientation=down  Expr=fc_inertia*(u*fd_ratio/wh_radius)^2
  veh mass calc : Subsystem
      settings: RTWFcnNameOpts=Auto  RTWFileNameOpts=Auto
  Out1 : Outport  Orientation=down  Port=1
  wires:
  [gear_ratio] -> engine inertia as a fraction of total vehicle inertia  (generous approximation)--numerator/1, engine inertia as a fraction of total vehicle inertia  (generous approximation)--denomenator/1
  veh mass calc/1(Out1) -> Sum/1
  engine inertia as a fraction of total vehicle inertia  (generous approximation)--denomenator/1 -> Sum/2
  engine inertia as a fraction of total vehicle inertia  (generous approximation)--numerator/1 -> Product/1
  Sum/1 -> Product/2
  Product/1 -> Out1/1

== system BD_CONV2/gearbox <gb> old/gearbox model & interface/gearbox model/Pout/Pin neglecting inertia/make division bombproof/Block NOTES ==
  note: this block added 10 July 2001 by mpo:
      | originally a -eps was added to the denominator by default.
      | However, cases were ecountered where Tin-Tineratia was equal to -eps causing
      | the denominator to be zero. This added checking is more rhobust

== system BD_CONV2/<cs> control strategy/Gearbox Control manual shift logic/manual shift logic/gearbox  control/shifting1/time since last shift/just shifted ==
  in_1 : Inport  Port=1  LatchInput=off
  Memory : Memory  X0=1  InheritSampleTime=off
      settings: RTWStateStorageClass=Auto
  Relational Operator : RelationalOperator  Operator=~=
  out_1 : Outport  Port=1  InitialOutput=0
  wires:
  Relational Operator/1 -> out_1/1
  Memory/1 -> Relational Operator/1
  in_1/1 -> Relational Operator/2, Memory/1

== system BD_CONV2/<cs> control strategy/Gearbox Control manual shift logic/manual shift logic/gearbox  control/shifting1/time since last shift/timer ==
  trigger : Inport  Port=1  LatchInput=off
  Constant : Constant  Value=1
  Constant1 : Constant  Value=0
  Constant2 : Constant  Value=0
  Switch : Switch  Threshold=eps
  no-lag Reset Integrator : Subsystem  mask(No-lag Reset Integrator){@1=15}
      mask prompts: @1 "Initial Value"
      mask help: No-lag Reset Integrator
      mask init:
      | initval=@1;
      settings: RTWFcnNameOpts=Auto  RTWFileNameOpts=Auto
      mask Help: Integrates first input using Euler technique.\nAt the time step that input 2 <> zero,\noutput is reset to input 3.
      mask Display: disp('1/s\nw/ reset\nno lag')
  time : Outport  Port=1  InitialOutput=0
  wires:
  Switch/1 -> time/1
  trigger/1 -> Switch/2, no-lag Reset Integrator/2(in_2)
  Constant2/1 -> Switch/1
  Constant/1 -> no-lag Reset Integrator/1(in_1)
  Constant1/1 -> no-lag Reset Integrator/3(in_3)
  no-lag Reset Integrator/1(out_1) -> Switch/3

== system BD_CONV2/fuel converter <fc>/IC Engine Model  &  Interface/ic engine model/engine torque/effect of inertia (Nm)/engine inertia as a function of total vehicle inertia (generous approximation)/veh mass calc ==
  Out1 : Outport  Port=1
  wires:
  [current_veh_mass] -> Out1/1

== system BD_CONV2/<cs> control strategy/Gearbox Control manual shift logic/manual shift logic/gearbox  control/shifting1/time since last shift/timer/no-lag Reset Integrator ==
  in_1 : Inport  Port=1  LatchInput=off
  in_2 : Inport  Port=2  LatchInput=off
  in_3 : Inport  Port=3  LatchInput=off
  Constant : Constant  Orientation=up  Value=0
  Memory : Memory  Orientation=left  X0=initval  InheritSampleTime=off
      settings: RTWStateStorageClass=Auto
  Product : Product  Inputs=2  Multiplication=Element-wise(.*)  SaturateOnIntegerOverflow=on
  Sum : Sum  Inputs=++  SaturateOnIntegerOverflow=on
  Switch : Switch  Threshold=eps
  dt : Subsystem  Orientation=down
      settings: RTWFcnNameOpts=Auto  RTWFileNameOpts=Auto
  in_2==0 : RelationalOperator  Operator===
  out_1 : Outport  Port=1  InitialOutput=0
  wires:
  Constant/1 -> in_2==0/2
  in_2==0/1 -> Switch/2
  Switch/1 -> Memory/1, out_1/1
  Sum/1 -> Switch/1
  Memory/1 -> Sum/1
  Product/1 -> Sum/2
  dt/1(out_1) -> Product/1
  in_1/1 -> Product/2
  in_2/1 -> in_2==0/1
  in_3/1 -> Switch/3

== system BD_CONV2/<cs> control strategy/Gearbox Control manual shift logic/manual shift logic/gearbox  control/shifting1/time since last shift/timer/no-lag Reset Integrator/dt ==
  Clock : Clock
      settings: DisplayTime=off  Decimation=10
  Memory1 : Memory  X0=-1  InheritSampleTime=off
      settings: RTWStateStorageClass=Auto
  Sum1 : Sum  Inputs=+-  SaturateOnIntegerOverflow=on
  out_1 : Outport  Port=1  InitialOutput=0
  wires:
  Sum1/1 -> out_1/1
  Memory1/1 -> Sum1/2
  Clock/1 -> Memory1/1, Sum1/1
